simulink model "onboard_SSC_simscape"  (R2025b)
settings: Solver=ode23t  StartTime=0.0  StopTime=0.5  RelTol=1e-3
undefined symbols (not defined in the file): Second_OrderFilter_class, Vbat_ref
libraries: fl_lib x28, nesl_utility x14, ee_lib x8, mcbeeMathTransformLib x3, slpidlib x1, eeGeneralControl x1, batteryecm_lib x1, eeSinusoidalMeasurementV2 x1, simulink x1
(part 1 of 2)
settings Model: SimulationMode=accelerator  Creator=zxd3816  LastModifiedBy=agarcian
settings SolverCC: AlgebraicLoopSolver=TrustRegion
settings DataIOCC: SignalLogging=off  DSMLogging=off  ReturnWorkspaceOutputs=off
settings DebuggingCC: SaveWithParameterizedLinksMsg=none  UnconnectedInputMsg=warning  UnconnectedOutputMsg=warning  UnconnectedLineMsg=warning
settings ModelReferenceCC: EnableRefExpFcnMdlSchedulingChecks=on
settings RTWCC: GPUComputeCapability=3.5  DLArmComputeVersion=19.05

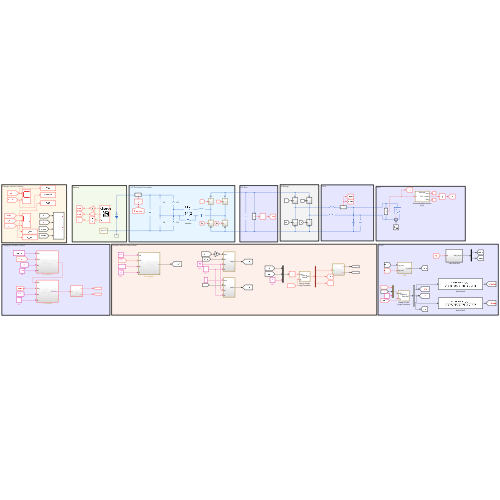
[thumbnail: Simulink's stored preview of the top-level diagram]
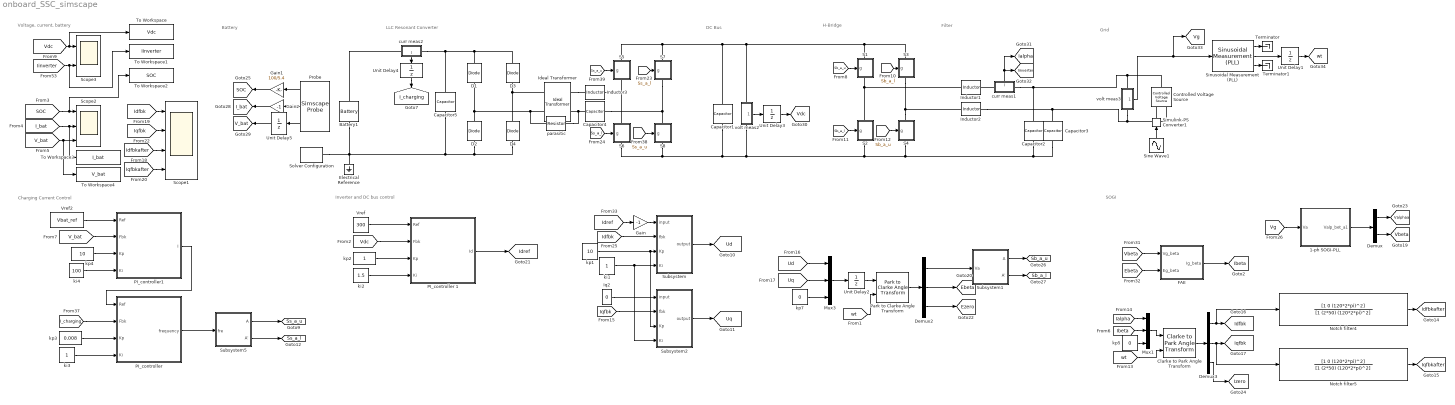
== system onboard_SSC_simscape ==
  note: Battery
  note: LLC Resonant Converter
  note: Charging Current Control
  note: SOGI
  note: Voltage, current, battery
  note: Inverter and DC bus control
  note: H-Bridge
  note: Filter
  note: DC Bus
  note: Grid
  1-ph SOGI-PLL : Subsystem
  Battery1 : batteryecm_lib/Battery  Vnom=100 V  prm_dir=simscape.enum.battery.prm_dir.disabled  R1_dis=2 Ohm  R1_ch=2 Ohm  R1=2 Ohm  prm_AH=simscape.enum.battery.prm_AH.finite  AH=5.4 A*hr  V1=95 V  AH1=0.54 A*hr  prm_R2=simscape.enum.battery.prm_R2.disabled  R2=2000 Ohm  Tmeas=298.15 K  charge_measurement_port=simscape.enum.battery.enable.no  prm_dyn=simscape.enum.battery.prm_dyn.off  Rp1=0.005 Ohm  tau1=30 s  Rp2=0.005 Ohm  tau2=30 s  Rp3=0.005 Ohm  tau3=30 s  Rp4=0.005 Ohm  tau4=30 s  Rp5=0.005 Ohm  tau5=30 s  prm_fade=simscape.enum.battery.prm_fade.disabled  N_fade=100  AH_fade=45 A*hr  R1_fade=2.02 Ohm  R1_ch_fade=2.02 Ohm  V1_fade=10.35 V  prm_age=simscape.enum.battery.prm_age.disabled  prm_age_OCV=simscape.enum.battery.prm_age_OCV.OCV  OCV_age=0.9  SOC_age=60  Tmeas_age=298.15 K  delta_time_age_vec=[0] d  temperature_age_vec=[273] K  OCV_scaling_age=2.2134e6  OCV_offset_age=1.632e6  temp_exp_age=0.515833569 V  t_exp_age=0.75  Vnom_T2=12 V  R1_T2=2.2 Ohm  R1_T2_dis=2.2 Ohm  R1_T2_ch=2.2 Ohm  V1_T2=11.4 V  R2_T2=2200 Ohm  Rp1_T2=0.005 Ohm  tau1_T2=30 s  Rp2_T2=0.005 Ohm  tau2_T2=30 s  Rp3_T2=0.005 Ohm  tau3_T2=30 s  Rp4_T2=0.005 Ohm  tau4_T2=30 s  Rp5_T2=0.005 Ohm  tau5_T2=30 s  Tmeas2=273.15 K  thermal_port=simscape.enum.thermaleffects.omit  thermal_mass=30000 J/K  i_specify=off  i_priority=None  i=0 A  i_nominal_specify=off  i_nominal_value=1  i_nominal_unit=A  v_specify=off  v_priority=None  v=0 V  v_nominal_specify=off  v_nominal_value=1  v_nominal_unit=V  charge_specify=on  charge_priority=High  charge=0.54 A*hr  charge_nominal_specify=off  charge_nominal_value=1  charge_nominal_unit=A*hr  num_cycles_specify=off  num_cycles_priority=High  num_cycles=0  num_cycles_nominal_specify=off  num_cycles_nominal_value=1  num_cycles_nominal_unit=1  temperature_specify=off  temperature_priority=High  temperature=298.15 K  temperature_nominal_specify=off  temperature_nominal_value=1  temperature_nominal_unit=K
  Capacitor1 : fl_lib/Electrical/Electrical Elements/Capacitor  c=500e-5 F  r=1e-9 Ohm  g=0 1/Ohm  i_specify=off  i_priority=None  i=0 A  i_nominal_specify=off  i_nominal_value=1  i_nominal_unit=A  v_specify=off  v_priority=None  v=0 V  v_nominal_specify=off  v_nominal_value=1  v_nominal_unit=V  vc_specify=off  vc_priority=High  vc=0 V  vc_nominal_specify=off  vc_nominal_value=1  vc_nominal_unit=V
  Capacitor2 : fl_lib/Electrical/Electrical Elements/Capacitor  c=60e-6 F  r=1e-9 Ohm  g=0 1/Ohm  i_specify=off  i_priority=None  i=0 A  i_nominal_specify=off  i_nominal_value=1  i_nominal_unit=A  v_specify=off  v_priority=None  v=0 V  v_nominal_specify=off  v_nominal_value=1  v_nominal_unit=V  vc_specify=off  vc_priority=High  vc=0 V  vc_nominal_specify=off  vc_nominal_value=1  vc_nominal_unit=V
  Capacitor3 : fl_lib/Electrical/Electrical Elements/Capacitor  c=60e-6 F  r=1e-9 Ohm  g=0 1/Ohm  i_specify=off  i_priority=None  i=0 A  i_nominal_specify=off  i_nominal_value=1  i_nominal_unit=A  v_specify=off  v_priority=None  v=0 V  v_nominal_specify=off  v_nominal_value=1  v_nominal_unit=V  vc_specify=off  vc_priority=High  vc=0 V  vc_nominal_specify=off  vc_nominal_value=1  vc_nominal_unit=V
  Capacitor4 : fl_lib/Electrical/Electrical Elements/Capacitor  c=110e-9 F  r=1e-6 Ohm  g=0 1/Ohm  i_specify=off  i_priority=None  i=0 A  i_nominal_specify=off  i_nominal_value=1  i_nominal_unit=A  v_specify=off  v_priority=None  v=0 V  v_nominal_specify=off  v_nominal_value=1  v_nominal_unit=V  vc_specify=off  vc_priority=High  vc=0 V  vc_nominal_specify=off  vc_nominal_value=1  vc_nominal_unit=V
  Capacitor5 : fl_lib/Electrical/Electrical Elements/Capacitor  c=500e-6 F  r=0 Ohm  g=0 1/Ohm  i_specify=off  i_priority=None  i=0 A  i_nominal_specify=off  i_nominal_value=1  i_nominal_unit=A  v_specify=off  v_priority=None  v=0 V  v_nominal_specify=off  v_nominal_value=1  v_nominal_unit=V  vc_specify=off  vc_priority=High  vc=0 V  vc_nominal_specify=off  vc_nominal_value=1  vc_nominal_unit=V
  Clarke to Park Angle Transform : mcbeeMathTransformLib/Clarke to Park Angle Transform  AxisAlignment=Q-axis  UseWithEmbedded=off  PhaseInput=Two inputs  ThetaInput=Sine and Cosine electrical position  AngleInput=Per-unit  N_points=1024
      settings: LibrarySourceBlock=|
      | ee_sl_lib/Mathematical
      | Transforms/Clarke to Park
      | Angle Transform
  Controlled Voltage Source : fl_lib/Electrical/Electrical Sources/Controlled Voltage Source
  D{1..4} (4 alike) : fl_lib/Electrical/Electrical Elements/Diode  Vf=0.8 V  Ron=0.001 Ohm  Goff=1/500 1/Ohm  i_specify=off  i_priority=None  i=0 A  i_nominal_specify=off  i_nominal_value=1  i_nominal_unit=A  v_specify=off  v_priority=None  v=0 V  v_nominal_specify=off  v_nominal_value=1  v_nominal_unit=V
  Demux : Demux  Outputs=2
  Demux2 : Demux  Outputs=3
  Demux3 : Demux  Outputs=3
  Electrical Reference : fl_lib/Electrical/Electrical Elements/Electrical Reference
  FAE : Subsystem
  Gain : Gain  Gain=-1
  Gain1 : Gain  Gain=100/5.4
  Gain2 : Gain  Gain=-1
  Ideal Transformer : fl_lib/Electrical/Electrical Elements/Ideal Transformer  n=1  i1_specify=off  i1_priority=None  i1=0 A  i1_nominal_specify=off  i1_nominal_value=1  i1_nominal_unit=A  v1_specify=off  v1_priority=None  v1=0 V  v1_nominal_specify=off  v1_nominal_value=1  v1_nominal_unit=V  i2_specify=off  i2_priority=None  i2=0 A  i2_nominal_specify=off  i2_nominal_value=1  i2_nominal_unit=A  v2_specify=off  v2_priority=None  v2=0 V  v2_nominal_specify=off  v2_nominal_value=1  v2_nominal_unit=V
  Inductor1 : fl_lib/Electrical/Electrical Elements/Inductor  l=3e-3 H  r=0.012 Ohm  g=0 1/Ohm  i_specify=off  i_priority=None  i=0 A  i_nominal_specify=off  i_nominal_value=1  i_nominal_unit=A  v_specify=off  v_priority=None  v=0 V  v_nominal_specify=off  v_nominal_value=1  v_nominal_unit=V  i_L_specify=off  i_L_priority=High  i_L=0 A  i_L_nominal_specify=off  i_L_nominal_value=1  i_L_nominal_unit=A
  Inductor2 : fl_lib/Electrical/Electrical Elements/Inductor  l=3e-3 H  r=0.012 Ohm  g=0 1/Ohm  i_specify=off  i_priority=None  i=0 A  i_nominal_specify=off  i_nominal_value=1  i_nominal_unit=A  v_specify=off  v_priority=None  v=0 V  v_nominal_specify=off  v_nominal_value=1  v_nominal_unit=V  i_L_specify=off  i_L_priority=High  i_L=0 A  i_L_nominal_specify=off  i_L_nominal_value=1  i_L_nominal_unit=A
  Inductor3 : fl_lib/Electrical/Electrical Elements/Inductor  l=21e-6 H  r=1e-6 Ohm  g=0 1/Ohm  i_specify=off  i_priority=None  i=0 A  i_nominal_specify=off  i_nominal_value=1  i_nominal_unit=A  v_specify=off  v_priority=None  v=0 V  v_nominal_specify=off  v_nominal_value=1  v_nominal_unit=V  i_L_specify=off  i_L_priority=High  i_L=0 A  i_L_nominal_specify=off  i_L_nominal_value=1  i_L_nominal_unit=A
  Iq2 : Constant  Value=0
  Mux1 : Mux  Inputs=3
  Mux3 : Mux  Inputs=3
  Notch filter4 : TransferFcn  Numerator=[1 0 (120*2*pi)^2]  Denominator=[1 (2*50) (120*2*pi)^2]
  Notch filter5 : TransferFcn  Numerator=[1 0 (120*2*pi)^2]  Denominator=[1 (2*50) (120*2*pi)^2]
  PI_controller : Subsystem
  PI_controller 1 : Subsystem
  PI_controller1 : Subsystem
  Park to Clarke Angle Transform : mcbeeMathTransformLib/Park to Clarke Angle Transform  AxisAlignment=Q-axis  UseWithEmbedded=off  PhaseInput=Two inputs  ThetaInput=Sine and Cosine electrical position  AngleInput=Per-unit  N_points=1024
      settings: LibrarySourceBlock=|
      | ee_sl_lib/Mathematical
      | Transforms/Park to Clarke
      | Angle Transform
  Probe : SimscapeProbe  BoundBlock=1503  Variables="{\"charge\":{\"Probing\":\"ON\"},\"i\":{\"Probing\":\"ON\"},\"v\":{\"Probing\":\"ON\"}}"
  S1 : Subsystem
      settings: PortSchema="{\"entries\":[{\"content\":{\"sides\":[{\"content\":{\"connectorIds\":[\"In1\"]},\"type\":\"ConnectorPlacement.EquallySpacedRectSide\",\"uuid\":\"60fc8352-b056-4a1d-84e9-807da1ce3c88\"},{\"content\":{\"side\":\"RIGHT\"},\"type\":\"ConnectorPlacement.EquallySpacedRectSide\",\"uuid\":\"4f85bb6a-64c7-4bda-b651-7e84ba390faf\"},{\"content\":{\"connectorIds\":[\"LConn1\"],\"side\":\"TOP\"},\"type\":\"ConnectorPlacement.EquallySpacedRectSide\",\"uuid\":\"49a2dfe1-7dda-4371-a15a-7ad00d7eb6fd\"},{\"content\":{\"connectorIds\":[\"RConn1\"],\"side\":\"BOTTOM\"},\"type\":\"ConnectorPlacement.EquallySpacedRectSide\",\"uuid\":\"2b076144-f23a-4c54-b109-69957c2c042c\"}]},\"type\":\"ConnectorPlacement.EquallySpacedConnector\",\"uuid\":\"c494b7b1-a248-4760-aec7-aedba1239c75\"}],\"packageUris\":[\"http://schema.mathworks.com/mf0/Connector/R2020b\"],\"version\":\"1.0\"}"
  S2 : Subsystem
      settings: PortSchema="{\"entries\":[{\"content\":{\"sides\":[{\"content\":{\"connectorIds\":[\"In1\"]},\"type\":\"ConnectorPlacement.EquallySpacedRectSide\",\"uuid\":\"60fc8352-b056-4a1d-84e9-807da1ce3c88\"},{\"content\":{\"side\":\"RIGHT\"},\"type\":\"ConnectorPlacement.EquallySpacedRectSide\",\"uuid\":\"4f85bb6a-64c7-4bda-b651-7e84ba390faf\"},{\"content\":{\"connectorIds\":[\"LConn1\"],\"side\":\"TOP\"},\"type\":\"ConnectorPlacement.EquallySpacedRectSide\",\"uuid\":\"49a2dfe1-7dda-4371-a15a-7ad00d7eb6fd\"},{\"content\":{\"connectorIds\":[\"RConn1\"],\"side\":\"BOTTOM\"},\"type\":\"ConnectorPlacement.EquallySpacedRectSide\",\"uuid\":\"2b076144-f23a-4c54-b109-69957c2c042c\"}]},\"type\":\"ConnectorPlacement.EquallySpacedConnector\",\"uuid\":\"c494b7b1-a248-4760-aec7-aedba1239c75\"}],\"packageUris\":[\"http://schema.mathworks.com/mf0/Connector/R2020b\"],\"version\":\"1.0\"}"
  S3 : Subsystem
      settings: PortSchema="{\"entries\":[{\"content\":{\"sides\":[{\"content\":{\"connectorIds\":[\"In1\"]},\"type\":\"ConnectorPlacement.EquallySpacedRectSide\",\"uuid\":\"60fc8352-b056-4a1d-84e9-807da1ce3c88\"},{\"content\":{\"side\":\"RIGHT\"},\"type\":\"ConnectorPlacement.EquallySpacedRectSide\",\"uuid\":\"4f85bb6a-64c7-4bda-b651-7e84ba390faf\"},{\"content\":{\"connectorIds\":[\"LConn1\"],\"side\":\"TOP\"},\"type\":\"ConnectorPlacement.EquallySpacedRectSide\",\"uuid\":\"49a2dfe1-7dda-4371-a15a-7ad00d7eb6fd\"},{\"content\":{\"connectorIds\":[\"RConn1\"],\"side\":\"BOTTOM\"},\"type\":\"ConnectorPlacement.EquallySpacedRectSide\",\"uuid\":\"2b076144-f23a-4c54-b109-69957c2c042c\"}]},\"type\":\"ConnectorPlacement.EquallySpacedConnector\",\"uuid\":\"c494b7b1-a248-4760-aec7-aedba1239c75\"}],\"packageUris\":[\"http://schema.mathworks.com/mf0/Connector/R2020b\"],\"version\":\"1.0\"}"
  S4 : Subsystem
      settings: PortSchema="{\"entries\":[{\"content\":{\"sides\":[{\"content\":{\"connectorIds\":[\"In1\"]},\"type\":\"ConnectorPlacement.EquallySpacedRectSide\",\"uuid\":\"60fc8352-b056-4a1d-84e9-807da1ce3c88\"},{\"content\":{\"side\":\"RIGHT\"},\"type\":\"ConnectorPlacement.EquallySpacedRectSide\",\"uuid\":\"4f85bb6a-64c7-4bda-b651-7e84ba390faf\"},{\"content\":{\"connectorIds\":[\"LConn1\"],\"side\":\"TOP\"},\"type\":\"ConnectorPlacement.EquallySpacedRectSide\",\"uuid\":\"49a2dfe1-7dda-4371-a15a-7ad00d7eb6fd\"},{\"content\":{\"connectorIds\":[\"RConn1\"],\"side\":\"BOTTOM\"},\"type\":\"ConnectorPlacement.EquallySpacedRectSide\",\"uuid\":\"2b076144-f23a-4c54-b109-69957c2c042c\"}]},\"type\":\"ConnectorPlacement.EquallySpacedConnector\",\"uuid\":\"c494b7b1-a248-4760-aec7-aedba1239c75\"}],\"packageUris\":[\"http://schema.mathworks.com/mf0/Connector/R2020b\"],\"version\":\"1.0\"}"
  S5 : Subsystem
      settings: PortSchema="{\"entries\":[{\"content\":{\"sides\":[{\"content\":{\"connectorIds\":[\"In1\"]},\"type\":\"ConnectorPlacement.EquallySpacedRectSide\",\"uuid\":\"60fc8352-b056-4a1d-84e9-807da1ce3c88\"},{\"content\":{\"side\":\"RIGHT\"},\"type\":\"ConnectorPlacement.EquallySpacedRectSide\",\"uuid\":\"4f85bb6a-64c7-4bda-b651-7e84ba390faf\"},{\"content\":{\"connectorIds\":[\"LConn1\"],\"side\":\"TOP\"},\"type\":\"ConnectorPlacement.EquallySpacedRectSide\",\"uuid\":\"49a2dfe1-7dda-4371-a15a-7ad00d7eb6fd\"},{\"content\":{\"connectorIds\":[\"RConn1\"],\"side\":\"BOTTOM\"},\"type\":\"ConnectorPlacement.EquallySpacedRectSide\",\"uuid\":\"2b076144-f23a-4c54-b109-69957c2c042c\"}]},\"type\":\"ConnectorPlacement.EquallySpacedConnector\",\"uuid\":\"c494b7b1-a248-4760-aec7-aedba1239c75\"}],\"packageUris\":[\"http://schema.mathworks.com/mf0/Connector/R2020b\"],\"version\":\"1.0\"}"
  S6 : Subsystem
      settings: PortSchema="{\"entries\":[{\"content\":{\"sides\":[{\"content\":{\"connectorIds\":[\"In1\"]},\"type\":\"ConnectorPlacement.EquallySpacedRectSide\",\"uuid\":\"60fc8352-b056-4a1d-84e9-807da1ce3c88\"},{\"content\":{\"side\":\"RIGHT\"},\"type\":\"ConnectorPlacement.EquallySpacedRectSide\",\"uuid\":\"4f85bb6a-64c7-4bda-b651-7e84ba390faf\"},{\"content\":{\"connectorIds\":[\"LConn1\"],\"side\":\"TOP\"},\"type\":\"ConnectorPlacement.EquallySpacedRectSide\",\"uuid\":\"49a2dfe1-7dda-4371-a15a-7ad00d7eb6fd\"},{\"content\":{\"connectorIds\":[\"RConn1\"],\"side\":\"BOTTOM\"},\"type\":\"ConnectorPlacement.EquallySpacedRectSide\",\"uuid\":\"2b076144-f23a-4c54-b109-69957c2c042c\"}]},\"type\":\"ConnectorPlacement.EquallySpacedConnector\",\"uuid\":\"c494b7b1-a248-4760-aec7-aedba1239c75\"}],\"packageUris\":[\"http://schema.mathworks.com/mf0/Connector/R2020b\"],\"version\":\"1.0\"}"
  S7 : Subsystem
      settings: PortSchema="{\"entries\":[{\"content\":{\"sides\":[{\"content\":{\"connectorIds\":[\"In1\"]},\"type\":\"ConnectorPlacement.EquallySpacedRectSide\",\"uuid\":\"60fc8352-b056-4a1d-84e9-807da1ce3c88\"},{\"content\":{\"side\":\"RIGHT\"},\"type\":\"ConnectorPlacement.EquallySpacedRectSide\",\"uuid\":\"4f85bb6a-64c7-4bda-b651-7e84ba390faf\"},{\"content\":{\"connectorIds\":[\"LConn1\"],\"side\":\"TOP\"},\"type\":\"ConnectorPlacement.EquallySpacedRectSide\",\"uuid\":\"49a2dfe1-7dda-4371-a15a-7ad00d7eb6fd\"},{\"content\":{\"connectorIds\":[\"RConn1\"],\"side\":\"BOTTOM\"},\"type\":\"ConnectorPlacement.EquallySpacedRectSide\",\"uuid\":\"2b076144-f23a-4c54-b109-69957c2c042c\"}]},\"type\":\"ConnectorPlacement.EquallySpacedConnector\",\"uuid\":\"c494b7b1-a248-4760-aec7-aedba1239c75\"}],\"packageUris\":[\"http://schema.mathworks.com/mf0/Connector/R2020b\"],\"version\":\"1.0\"}"
  S8 : Subsystem
      settings: PortSchema="{\"entries\":[{\"content\":{\"sides\":[{\"content\":{\"connectorIds\":[\"In1\"]},\"type\":\"ConnectorPlacement.EquallySpacedRectSide\",\"uuid\":\"60fc8352-b056-4a1d-84e9-807da1ce3c88\"},{\"content\":{\"side\":\"RIGHT\"},\"type\":\"ConnectorPlacement.EquallySpacedRectSide\",\"uuid\":\"4f85bb6a-64c7-4bda-b651-7e84ba390faf\"},{\"content\":{\"connectorIds\":[\"LConn1\"],\"side\":\"TOP\"},\"type\":\"ConnectorPlacement.EquallySpacedRectSide\",\"uuid\":\"49a2dfe1-7dda-4371-a15a-7ad00d7eb6fd\"},{\"content\":{\"connectorIds\":[\"RConn1\"],\"side\":\"BOTTOM\"},\"type\":\"ConnectorPlacement.EquallySpacedRectSide\",\"uuid\":\"2b076144-f23a-4c54-b109-69957c2c042c\"}]},\"type\":\"ConnectorPlacement.EquallySpacedConnector\",\"uuid\":\"c494b7b1-a248-4760-aec7-aedba1239c75\"}],\"packageUris\":[\"http://schema.mathworks.com/mf0/Connector/R2020b\"],\"version\":\"1.0\"}"
  Scope1 : Scope  NumInputPorts=4
      settings: ActiveDisplayYMinimum=-174.13299  ActiveDisplayYMaximum=150.39718
  Scope2 : Scope  NumInputPorts=3
      settings: ActiveDisplayYMinimum=9.9934066794791612  ActiveDisplayYMaximum=10.056826198144963
  Scope3 : Scope  NumInputPorts=2
      settings: ActiveDisplayYMinimum=-38.68725  ActiveDisplayYMaximum=348.18522  DataLoggingVariableName=ScopeData3
  Simulink-PS Converter1 : nesl_utility/Simulink-PS Converter  PhysicalDomain=network_engine_domain  SubClassName=ps_input  LeftPortType=input  RightPortType=output  PseudoPeriodic=off  Frequencies=[]  NoiseDistribution=none  NoiseParameters=[]  Unit=1  AffineConversion=off  FilteringAndDerivatives=provide  SimscapeFilterOrder=1  InputFilterTimeConstant=0.001  UdotUserProvided=0
  Sine Wave1 : Sin  Amplitude=169.7  Frequency=60*2*pi  SampleTime=0
  Sinusoidal Measurement (PLL) : eeSinusoidalMeasurementV2/Sinusoidal Measurement (PLL)  Ki_PD=3200  Kp_LF=180  Ki_LF=3200  F0=60  Theta0=0  Mag0=1  Ts=-1
      settings: LibrarySourceBlock=|
      | ee_sl_lib/Measurements/Sinusoidal Measurement
      | (PLL)
  Solver Configuration : nesl_utility/Solver Configuration  PhysicalDomain=network_engine_domain  SubClassName=solver  LeftPortType=input  RightPortType=generic  Tones=[]  Harmonics=[]  SimulateNoise=off  Profile=off  UseLocalSampling=off  EnableSwitchedLinearOptims=on  FrequencyDomain=off  UseCCode=off  RelTol=0.001  AbsTol=0.001  MinStep=1e-09  ToWorkspace=off  RevertToSquareIcSolve=off  NumHomotopyIterations=100  PhasorMode=off  PhasorModeNumHarmonics=1  ConsistencySolver=NEWTON_XTOL_AFTER_FTOL  IndexReductionMethod=DerivativeReplacement  DoDC=off  ResidualTolerance=1e-09  ConsistencyTolSource=GLOBAL  ConsistencyAbsTol=0.001  ConsistencyRelTol=0.001  ConsistencyTolFactor=0.001  UseLocalSolver=on  LocalSolverChoice=NE_PARTITIONING_ADVANCER  ResolveIndetEquations=off  FunctionEvalNumThread=1  LocalSolverSampleTime=1e-7  DoFixedCost=off  MaxNonlinIter=2  MaxModeIter=2  ComputeImpulses=off  ImpulseIterations=2  LinearAlgebra=auto  LinearAlgebraNumThread=0  EquationFormulation=NE_TIME_EF  DelaysMemoryBudget=1024  AutomaticFiltering=off  FilteringTimeConstant=0.001  PartitionStorageMethod=AS_NEEDED  PartitionMemoryBudget=1024  PartitionMethod=ROBUST  MultibodyUseLocalSolver=off  MultibodyLocalSolverChoice=ODE1  MultibodyLocalSolverSampleTime=0.001
  Subsystem : Subsystem
  Subsystem1 : Subsystem
  Subsystem2 : Subsystem
  Subsystem5 : Subsystem
  Terminator : Terminator
  Terminator1 : Terminator
  To Workspace : ToWorkspace  VariableName=Vdc  SampleTime=-1
  To Workspace1 : ToWorkspace  VariableName=Iinverter  SampleTime=-1
  To Workspace2 : ToWorkspace  VariableName=SOC  SampleTime=-1
  To Workspace3 : ToWorkspace  VariableName=I_bat  SampleTime=-1
  To Workspace4 : ToWorkspace  VariableName=V_bat  SampleTime=-1
  Unit Delay{1..5} (5 alike) : UnitDelay  SampleTime=-1  HasFrameUpgradeWarning=on
  Vref : Constant  Value=300
  Vref2 : Constant  Value=Vbat_ref
  curr meas1 : Subsystem
      settings: PortSchema="{\"entries\":[{\"content\":{\"sides\":[{\"content\":{\"connectorIds\":[\"LConn1\"]},\"type\":\"ConnectorPlacement.EquallySpacedRectSide\",\"uuid\":\"624dd8c9-1efa-425a-b23f-9e7d392e4567\"},{\"content\":{\"connectorIds\":[\"RConn1\"],\"side\":\"RIGHT\"},\"type\":\"ConnectorPlacement.EquallySpacedRectSide\",\"uuid\":\"c564bb74-22a6-4c48-884d-57ae53c7e586\"},{\"content\":{\"connectorIds\":[\"Out1\"],\"side\":\"TOP\"},\"type\":\"ConnectorPlacement.EquallySpacedRectSide\",\"uuid\":\"df3a0756-8bf4-4498-aa4e-0bb1b4f3eded\"}]},\"type\":\"ConnectorPlacement.EquallySpacedConnector\",\"uuid\":\"9eff73ec-b3ab-492c-96fa-8ca694a66385\"}],\"packageUris\":[\"http://schema.mathworks.com/mf0/Connector/R2020b\"],\"version\":\"1.0\"}"
  curr meas2 : Subsystem
      settings: PortSchema="{\"entries\":[{\"content\":{\"sides\":[{\"content\":{\"connectorIds\":[\"LConn1\"]},\"type\":\"ConnectorPlacement.EquallySpacedRectSide\",\"uuid\":\"624dd8c9-1efa-425a-b23f-9e7d392e4567\"},{\"content\":{\"connectorIds\":[\"RConn1\"],\"side\":\"RIGHT\"},\"type\":\"ConnectorPlacement.EquallySpacedRectSide\",\"uuid\":\"c564bb74-22a6-4c48-884d-57ae53c7e586\"},{\"content\":{\"connectorIds\":[\"Out1\"],\"side\":\"TOP\"},\"type\":\"ConnectorPlacement.EquallySpacedRectSide\",\"uuid\":\"df3a0756-8bf4-4498-aa4e-0bb1b4f3eded\"}]},\"type\":\"ConnectorPlacement.EquallySpacedConnector\",\"uuid\":\"9eff73ec-b3ab-492c-96fa-8ca694a66385\"}],\"packageUris\":[\"http://schema.mathworks.com/mf0/Connector/R2020b\"],\"version\":\"1.0\"}"
  ki1 : Constant
  ki2 : Constant  Value=1.5
  ki3 : Constant
  ki4 : Constant  Value=100
  kp1 : Constant  Value=10
  kp2 : Constant
  kp3 : Constant  Value=0.008
  kp4 : Constant  Value=10
  kp5 : Constant  Value=0
  kp7 : Constant  Value=0
  parasitic : fl_lib/Electrical/Electrical Elements/Resistor  R=1e8 Ohm  i_specify=off  i_priority=None  i=0 A  i_nominal_specify=off  i_nominal_value=1  i_nominal_unit=A  v_specify=off  v_priority=None  v=0 V  v_nominal_specify=off  v_nominal_value=1  v_nominal_unit=V
  volt meas2 : Subsystem
      settings: PortSchema="{\"entries\":[{\"content\":{\"sides\":[{\"content\":{},\"type\":\"ConnectorPlacement.EquallySpacedRectSide\",\"uuid\":\"624dd8c9-1efa-425a-b23f-9e7d392e4567\"},{\"content\":{\"connectorIds\":[\"Out1\"],\"side\":\"RIGHT\"},\"type\":\"ConnectorPlacement.EquallySpacedRectSide\",\"uuid\":\"c564bb74-22a6-4c48-884d-57ae53c7e586\"},{\"content\":{\"connectorIds\":[\"LConn1\"],\"side\":\"TOP\"},\"type\":\"ConnectorPlacement.EquallySpacedRectSide\",\"uuid\":\"df3a0756-8bf4-4498-aa4e-0bb1b4f3eded\"},{\"content\":{\"connectorIds\":[\"RConn1\"],\"side\":\"BOTTOM\"},\"type\":\"ConnectorPlacement.EquallySpacedRectSide\",\"uuid\":\"6b8e9540-8d6f-4bd3-bf1f-20eb25478a8e\"}]},\"type\":\"ConnectorPlacement.EquallySpacedConnector\",\"uuid\":\"9eff73ec-b3ab-492c-96fa-8ca694a66385\"}],\"packageUris\":[\"http://schema.mathworks.com/mf0/Connector/R2020b\"],\"version\":\"1.0\"}"
  volt meas3 : Subsystem
      settings: PortSchema="{\"entries\":[{\"content\":{\"sides\":[{\"content\":{},\"type\":\"ConnectorPlacement.EquallySpacedRectSide\",\"uuid\":\"624dd8c9-1efa-425a-b23f-9e7d392e4567\"},{\"content\":{\"connectorIds\":[\"Out1\"],\"side\":\"RIGHT\"},\"type\":\"ConnectorPlacement.EquallySpacedRectSide\",\"uuid\":\"c564bb74-22a6-4c48-884d-57ae53c7e586\"},{\"content\":{\"connectorIds\":[\"LConn1\"],\"side\":\"TOP\"},\"type\":\"ConnectorPlacement.EquallySpacedRectSide\",\"uuid\":\"df3a0756-8bf4-4498-aa4e-0bb1b4f3eded\"},{\"content\":{\"connectorIds\":[\"RConn1\"],\"side\":\"BOTTOM\"},\"type\":\"ConnectorPlacement.EquallySpacedRectSide\",\"uuid\":\"6b8e9540-8d6f-4bd3-bf1f-20eb25478a8e\"}]},\"type\":\"ConnectorPlacement.EquallySpacedConnector\",\"uuid\":\"9eff73ec-b3ab-492c-96fa-8ca694a66385\"}],\"packageUris\":[\"http://schema.mathworks.com/mf0/Connector/R2020b\"],\"version\":\"1.0\"}"
  tag scope: Ebeta=global, Ezero=global, I_bat=global, I_charging=global, Ialpha=global, Ibeta=global, Idfbk=global, Idfbkafter=global, Idref=global, Iinverter=global, Iqfbk=global, Iqfbkafter=global, Izero=global, SOC=global, Sb_a_l=global, Sb_a_u=global, Ss_a_l=global, Ss_a_u=global, Ud=global, Uq=global, V_bat=global, Valphaa=global, Vbeta=global, Vdc=global, Vg=global, wt=global
  wires:
  [Iqfbk] -> Scope1/2
  [Idfbk] -> Scope1/1
  [Vdc] -> To Workspace/1, Scope3/1
  [Iinverter] -> To Workspace1/1, Scope3/2
  Demux2/3 -> [Ezero]
  Subsystem/1(output) -> [Ud]
  kp1/1 -> Subsystem2/3(Kp), Subsystem/3(Kp)
  Subsystem2/1(output) -> [Uq]
  ki1/1 -> Subsystem2/4(Ki), Subsystem/4(Ki)
  kp2/1 -> PI_controller 1/3(Kp)
  ki2/1 -> PI_controller 1/4(Ki)
  Vref/1 -> PI_controller 1/1(Ref)
  [Vdc] -> PI_controller 1/2(Fbk)
  Iq2/1 -> Subsystem2/1(input)
  [Iqfbk] -> Subsystem2/2(fbk)
  Demux2/1 -> Subsystem1/1(Va)
  [Idfbk] -> Subsystem/2(fbk)
  Mux3/1 -> Unit Delay2/1
  [Ud] -> Mux3/1
  [Uq] -> Mux3/2
  kp7/1 -> Mux3/3
  [wt] -> Park to Clarke Angle Transform/2
  Park to Clarke Angle Transform/1 -> Demux2/1
  Demux3/1 -> Notch filter4/1, [Idfbk]
  Notch filter4/1 -> [Idfbkafter]
  Clarke to Park Angle Transform/1 -> Demux3/1
  Notch filter5/1 -> [Iqfbkafter]
  [wt] -> Clarke to Park Angle Transform/2
  Demux3/2 -> Notch filter5/1, [Iqfbk]
  Mux1/1 -> Clarke to Park Angle Transform/1
  [Ialpha] -> Mux1/1
  1-ph SOGI-PLL/1(Valp_bet_a1) -> Demux/1
  FAE/1(Ig_beta) -> [Ibeta]
  [Ibeta] -> Mux1/2
  [Idfbkafter] -> Scope1/3
  [Iqfbkafter] -> Scope1/4
  [Vg] -> 1-ph SOGI-PLL/1(Va)
  Demux/2 -> [Vbeta]
  [Vbeta] -> FAE/1(Vg_beta)
  Demux2/2 -> [Ebeta]
  [Ebeta] -> FAE/2(Eg_beta)
  PI_controller 1/1(Id) -> [Idref]
  Demux/1 -> [Valphaa]
  Demux3/3 -> [Izero]
  Gain/1 -> Subsystem/1(input)
  Subsystem1/1(A) -> [Sb_a_u]
  Subsystem1/2(A') -> [Sb_a_l]
  [Idref] -> Gain/1
  Subsystem5/1(A) -> [Ss_a_u]
  Subsystem5/2(A') -> [Ss_a_l]
  PI_controller/1(frequency) -> Subsystem5/1(fre)
  kp3/1 -> PI_controller/3(Kp)
  ki3/1 -> PI_controller/4(Ki)
  [I_charging] -> PI_controller/2(Fbk)
  [SOC] -> To Workspace2/1, Scope2/1
  [I_bat] -> To Workspace3/1, Scope2/2
  [V_bat] -> To Workspace4/1, Scope2/3
  Vref2/1 -> PI_controller1/1(Ref)
  [V_bat] -> PI_controller1/2(Fbk)
  kp4/1 -> PI_controller1/3(Kp)
  ki4/1 -> PI_controller1/4(Ki)
  PI_controller1/1(I) -> PI_controller/1(Ref)
  volt meas2/1(V) -> Unit Delay3/1
  Sinusoidal Measurement (PLL)/2 -> Unit Delay1/1
  Sinusoidal Measurement (PLL)/1 -> Terminator/1
  Unit Delay3/1 -> [Vdc]
  [Sb_a_u] -> S4/1(g)
  curr meas1/1(I) -> [Iinverter], [Ialpha]
  Sinusoidal Measurement (PLL)/3 -> Terminator1/1
  [Sb_a_u] -> S1/1(g)
  [Sb_a_l] -> S3/1(g)
  Unit Delay1/1 -> [wt]
  Sine Wave1/1 -> Simulink-PS Converter1/1
  volt meas3/1(V) -> Sinusoidal Measurement (PLL)/1, [Vg]
  [Sb_a_l] -> S2/1(g)
  [Ss_a_l] -> S6/1(g)
  [Ss_a_l] -> S7/1(g)
  [Ss_a_u] -> S5/1(g)
  [Ss_a_u] -> S8/1(g)
  curr meas2/1(I) -> Unit Delay4/1
  Probe/1 -> Gain1/1
  Probe/3 -> Unit Delay5/1
  Gain1/1 -> [SOC]
  kp5/1 -> Mux1/3
  Unit Delay2/1 -> Park to Clarke Angle Transform/1
  Unit Delay4/1 -> [I_charging]
  Unit Delay5/1 -> [V_bat]
  Probe/2 -> Gain2/1
  Gain2/1 -> [I_bat]
  connections:
  S7/LConn1 -- volt meas2/LConn1 -- S3/LConn1 -- S1/LConn1 -- Capacitor1/LConn1 -- S5/LConn1
  Capacitor2/RConn1 -- volt meas2/RConn1 -- Capacitor1/RConn1 -- S8/RConn1 -- S6/RConn1 -- S2/RConn1 -- S4/RConn1 -- Capacitor3/RConn1
  Capacitor2/LConn1 -- curr meas1/RConn1 -- Controlled Voltage Source/LConn1 -- volt meas3/LConn1
  Controlled Voltage Source/RConn2 -- volt meas3/RConn1 -- Inductor2/RConn1 -- Capacitor3/LConn1
  Inductor1/LConn1 -- S2/LConn1 -- S1/RConn1
  S4/LConn1 -- S3/RConn1 -- Inductor2/LConn1
  Simulink-PS Converter1/RConn1 -- Controlled Voltage Source/RConn1
  curr meas1/LConn1 -- Inductor1/RConn1
  Ideal Transformer/RConn1 -- Inductor3/LConn1
  Ideal Transformer/RConn2 -- parasitic/RConn1 -- Capacitor4/LConn1
  S6/LConn1 -- Inductor3/RConn1 -- S5/RConn1
  S7/RConn1 -- S8/LConn1 -- Capacitor4/RConn1
  D2/RConn1 -- parasitic/LConn1 -- Ideal Transformer/LConn2 -- D1/LConn1
  D4/RConn1 -- Ideal Transformer/LConn1 -- D3/LConn1
  D3/RConn1 -- Capacitor5/LConn1 -- curr meas2/LConn1 -- D1/RConn1
  D4/LConn1 -- D2/LConn1 -- Electrical Reference/LConn1 -- Battery1/RConn1 -- Solver Configuration/RConn1 -- Capacitor5/RConn1
  Battery1/LConn1 -- curr meas2/RConn1

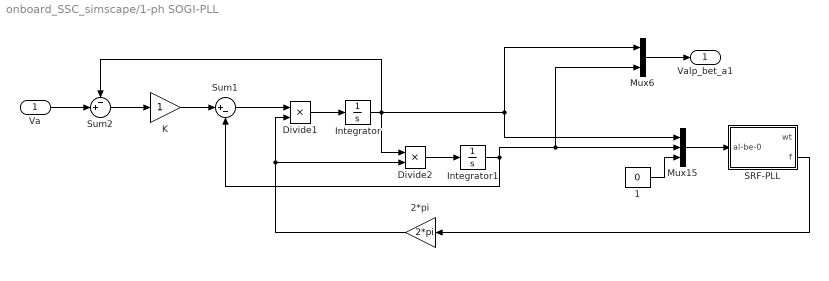
== system onboard_SSC_simscape/1-ph SOGI-PLL ==
  Va : Inport
  1 : Constant  Value=0
  2*pi : Gain  Gain=2*pi
  Divide1 : Product  Inputs=**
  Divide2 : Product  Inputs=**
  Integrator : Integrator
  Integrator1 : Integrator
  K : Gain
  Mux15 : Mux  Inputs=3
  Mux6 : Mux  Inputs=2
  SRF-PLL : Subsystem
  Sum1 : Sum  Inputs=|+-
  Sum2 : Sum  Inputs=-+|
  Valp_bet_a1 : Outport
  wires:
  Divide1/1 -> Integrator/1
  Sum1/1 -> Divide1/1
  K/1 -> Sum1/1
  Sum2/1 -> K/1
  Integrator/1 -> Sum2/1, Divide2/1, Mux15/1, Mux6/1
  Divide2/1 -> Integrator1/1
  Integrator1/1 -> Sum1/2, Mux6/2, Mux15/2
  Va/1 -> Sum2/2
  1/1 -> Mux15/3
  Mux15/1 -> SRF-PLL/1(al-be-0)
  2*pi/1 -> Divide2/2, Divide1/2
  SRF-PLL/2(f) -> 2*pi/1
  Mux6/1 -> Valp_bet_a1/1

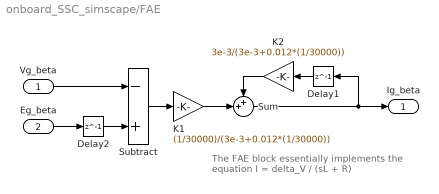
== system onboard_SSC_simscape/FAE ==
  note: The FAE block essentially implements the equation I = delta_V / (sL + R)
  Vg_beta : Inport
  Eg_beta : Inport  Port=2
  Delay1 : Delay  DelayLength=1
  Delay2 : Delay  DelayLength=1
  K1 : Gain  Gain=(1/30000)/(3e-3+0.012*(1/30000))
  K2 : Gain  Gain=3e-3/(3e-3+0.012*(1/30000))
  Subtract : Sum  Inputs=-+
  Sum : Sum  Inputs=++|
  Ig_beta : Outport
  wires:
  Eg_beta/1 -> Delay2/1
  Delay2/1 -> Subtract/2
  Sum/1 -> Ig_beta/1, Delay1/1
  K2/1 -> Sum/1
  Delay1/1 -> K2/1
  K1/1 -> Sum/2
  Subtract/1 -> K1/1
  Vg_beta/1 -> Subtract/1

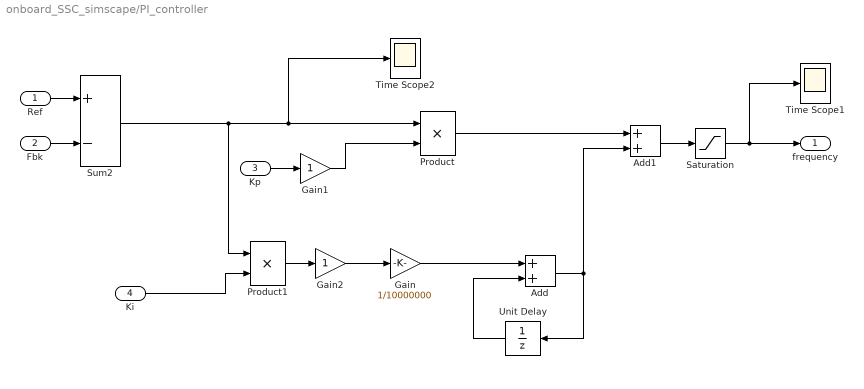
== system onboard_SSC_simscape/PI_controller ==
  Ref : Inport
  Fbk : Inport  Port=2
  Kp : Inport  Port=3
  Ki : Inport  Port=4
  Add : Sum
  Add1 : Sum
  Gain : Gain  Gain=1/10000000
  Gain1 : Gain
  Gain2 : Gain
  Product : Product  OutDataTypeStr=Inherit: Same as first input
  Product1 : Product  OutDataTypeStr=Inherit: Same as first input
  Saturation : Saturate  UpperLimit=1  LowerLimit=0.5  LinearizeAsGain=off  ZeroCross=off
  Sum2 : Sum  Inputs=+-
  Time Scope1 : Scope
      settings: TimeUnits=Metric (based on Time Span)  ActiveDisplayYMinimum=0.5433  ActiveDisplayYMaximum=1.0015  YLabel=Amplitude  DataLoggingVariableName=ScopeData5
  Time Scope2 : Scope
      settings: TimeUnits=Metric (based on Time Span)  ActiveDisplayYMinimum=-48.22028  ActiveDisplayYMaximum=227.58003  YLabel=Amplitude  DataLoggingVariableName=ScopeData6
  Unit Delay : UnitDelay  InitialCondition=0.9  SampleTime=-1  HasFrameUpgradeWarning=on
  frequency : Outport
  wires:
  Fbk/1 -> Sum2/2
  Ref/1 -> Sum2/1
  Product1/1 -> Gain2/1
  Add/1 -> Unit Delay/1, Add1/2
  Product/1 -> Add1/1
  Gain/1 -> Add/1
  Unit Delay/1 -> Add/2
  Ki/1 -> Product1/2
  Gain2/1 -> Gain/1
  Add1/1 -> Saturation/1
  Saturation/1 -> Time Scope1/1, frequency/1
  Kp/1 -> Gain1/1
  Gain1/1 -> Product/2
  Sum2/1 -> Product1/1, Time Scope2/1, Product/1

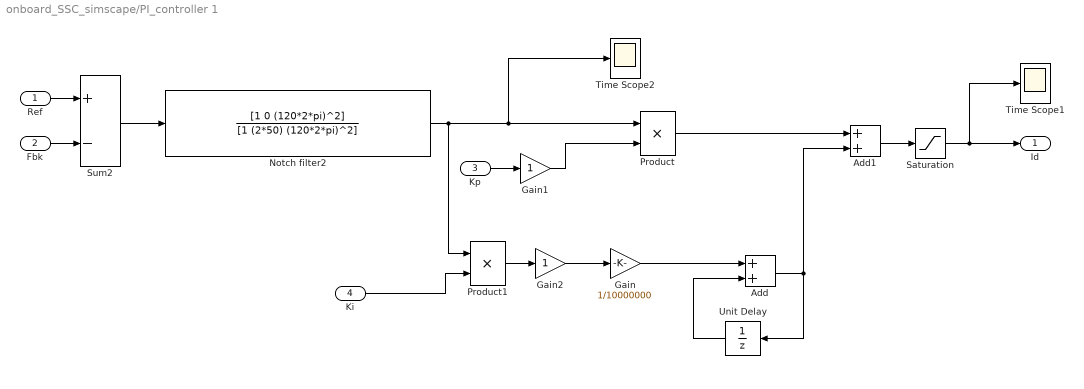
== system onboard_SSC_simscape/PI_controller 1 ==
  Ref : Inport
  Fbk : Inport  Port=2
  Kp : Inport  Port=3
  Ki : Inport  Port=4
  Add : Sum
  Add1 : Sum
  Gain : Gain  Gain=1/10000000
  Gain1 : Gain
  Gain2 : Gain
  Notch filter2 : TransferFcn  Numerator=[1 0 (120*2*pi)^2]  Denominator=[1 (2*50) (120*2*pi)^2]
  Product : Product  OutDataTypeStr=Inherit: Same as first input
  Product1 : Product  OutDataTypeStr=Inherit: Same as first input
  Saturation : Saturate  UpperLimit=100  LowerLimit=-100  LinearizeAsGain=off  ZeroCross=off
  Sum2 : Sum  Inputs=+-
  Time Scope1 : Scope
      settings: TimeUnits=Metric (based on Time Span)  ActiveDisplayYMinimum=-62.5  ActiveDisplayYMaximum=62.5  YLabel=Amplitude  DataLoggingVariableName=ScopeData5
  Time Scope2 : Scope
      settings: TimeUnits=Metric (based on Time Span)  ActiveDisplayYMinimum=-48.22028  ActiveDisplayYMaximum=227.58003  YLabel=Amplitude  DataLoggingVariableName=ScopeData6
  Unit Delay : UnitDelay  SampleTime=-1  HasFrameUpgradeWarning=on
  Id : Outport
  wires:
  Fbk/1 -> Sum2/2
  Ref/1 -> Sum2/1
  Product1/1 -> Gain2/1
  Add/1 -> Unit Delay/1, Add1/2
  Product/1 -> Add1/1
  Gain/1 -> Add/1
  Unit Delay/1 -> Add/2
  Ki/1 -> Product1/2
  Gain2/1 -> Gain/1
  Add1/1 -> Saturation/1
  Saturation/1 -> Time Scope1/1, Id/1
  Kp/1 -> Gain1/1
  Gain1/1 -> Product/2
  Sum2/1 -> Notch filter2/1
  Notch filter2/1 -> Product1/1, Time Scope2/1, Product/1

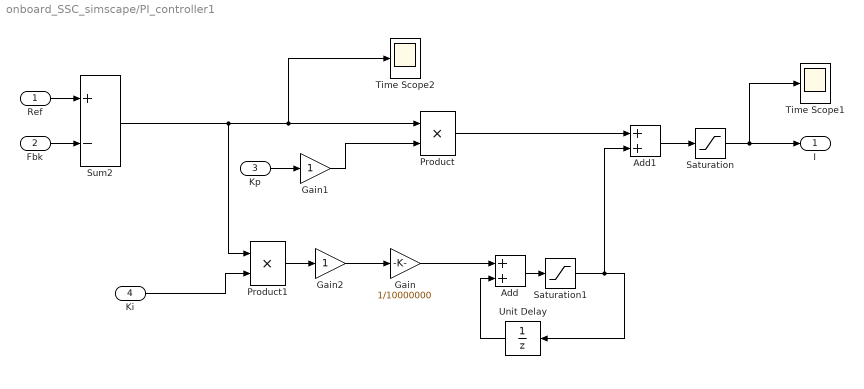
== system onboard_SSC_simscape/PI_controller1 ==
  Ref : Inport
  Fbk : Inport  Port=2
  Kp : Inport  Port=3
  Ki : Inport  Port=4
  Add : Sum
  Add1 : Sum
  Gain : Gain  Gain=1/10000000
  Gain1 : Gain
  Gain2 : Gain
  Product : Product  OutDataTypeStr=Inherit: Same as first input
  Product1 : Product  OutDataTypeStr=Inherit: Same as first input
  Saturation : Saturate  UpperLimit=20  LowerLimit=0  LinearizeAsGain=off  ZeroCross=off
  Saturation1 : Saturate  UpperLimit=30  LowerLimit=-30  LinearizeAsGain=off  ZeroCross=off
  Sum2 : Sum  Inputs=+-
  Time Scope1 : Scope
      settings: TimeUnits=Metric (based on Time Span)  ActiveDisplayYMinimum=10.50458  ActiveDisplayYMaximum=21.05505  YLabel=Amplitude  DataLoggingVariableName=ScopeData5
  Time Scope2 : Scope
      settings: TimeUnits=Metric (based on Time Span)  ActiveDisplayYMinimum=-48.22028  ActiveDisplayYMaximum=227.58003  YLabel=Amplitude  DataLoggingVariableName=ScopeData6
  Unit Delay : UnitDelay  InitialCondition=0.9  SampleTime=-1  HasFrameUpgradeWarning=on
  I : Outport
  wires:
  Fbk/1 -> Sum2/2
  Ref/1 -> Sum2/1
  Product1/1 -> Gain2/1
  Product/1 -> Add1/1
  Gain/1 -> Add/1
  Unit Delay/1 -> Add/2
  Ki/1 -> Product1/2
  Gain2/1 -> Gain/1
  Add1/1 -> Saturation/1
  Saturation/1 -> Time Scope1/1, I/1
  Kp/1 -> Gain1/1
  Gain1/1 -> Product/2
  Sum2/1 -> Product1/1, Time Scope2/1, Product/1
  Add/1 -> Saturation1/1
  Saturation1/1 -> Add1/2, Unit Delay/1

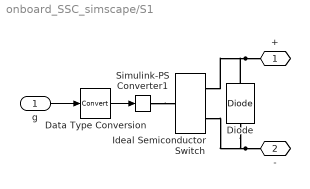
== system onboard_SSC_simscape/S1 ==
  g : Inport
  Data Type Conversion : DataTypeConversion  SaturateOnIntegerOverflow=off  RndMeth=Floor
  Diode : fl_lib/Electrical/Electrical Elements/Diode  Vf=1e-3 V  Ron=0.01 Ohm  Goff=1e-5 1/Ohm  i_specify=off  i_priority=None  i=0 A  i_nominal_specify=off  i_nominal_value=1  i_nominal_unit=A  v_specify=off  v_priority=None  v=0 V  v_nominal_specify=off  v_nominal_value=1  v_nominal_unit=V
  Ideal Semiconductor Switch : ee_lib/Semiconductors & Converters/Ideal Semiconductor Switch  port_option=ee.enum.controlport.ps  Ron=0.1 Ohm  Goff=1e-5 1/Ohm  Vth=0.5 V  diode_param=ee.enum.semiconductors.protectionDiode.external  diode_Vf=1e-3 V  diode_Ron=0.01 Ohm  diode_Goff=1e-5 1/Ohm  diode_C=50e-9 F  diode_iRM=-235 A  diode_iF=300 A  diode_idot=-50 A/us  diode_trr_param=ee.enum.converters.diodetrr.trr_factor  diode_trr_factor=3  diode_trr=15 us  diode_Qrr=1500 s*uA
  Simulink-PS Converter1 : nesl_utility/Simulink-PS Converter  PhysicalDomain=network_engine_domain  SubClassName=ps_input  LeftPortType=input  RightPortType=output  PseudoPeriodic=off  Frequencies=[]  NoiseDistribution=none  NoiseParameters=[]  Unit=1  AffineConversion=off  FilteringAndDerivatives=provide  SimscapeFilterOrder=1  InputFilterTimeConstant=0.001  UdotUserProvided=0
  + : PMIOPort  Side=Left
  - : PMIOPort  Port=2  Side=Right
  wires:
  Data Type Conversion/1 -> Simulink-PS Converter1/1
  g/1 -> Data Type Conversion/1
  connections:
  -/RConn1 -- Diode/LConn1 -- Ideal Semiconductor Switch/RConn2
  +/RConn1 -- Diode/RConn1 -- Ideal Semiconductor Switch/RConn1
  Simulink-PS Converter1/RConn1 -- Ideal Semiconductor Switch/LConn1

== system onboard_SSC_simscape/S2 ==
  g : Inport
  Data Type Conversion : DataTypeConversion  SaturateOnIntegerOverflow=off  RndMeth=Floor
  Diode : fl_lib/Electrical/Electrical Elements/Diode  Vf=1e-3 V  Ron=0.01 Ohm  Goff=1e-5 1/Ohm  i_specify=off  i_priority=None  i=0 A  i_nominal_specify=off  i_nominal_value=1  i_nominal_unit=A  v_specify=off  v_priority=None  v=0 V  v_nominal_specify=off  v_nominal_value=1  v_nominal_unit=V
  Ideal Semiconductor Switch : ee_lib/Semiconductors & Converters/Ideal Semiconductor Switch  port_option=ee.enum.controlport.ps  Ron=0.1 Ohm  Goff=1e-5 1/Ohm  Vth=0.5 V  diode_param=ee.enum.semiconductors.protectionDiode.external  diode_Vf=1e-3 V  diode_Ron=0.01 Ohm  diode_Goff=1e-5 1/Ohm  diode_C=50e-9 F  diode_iRM=-235 A  diode_iF=300 A  diode_idot=-50 A/us  diode_trr_param=ee.enum.converters.diodetrr.trr_factor  diode_trr_factor=3  diode_trr=15 us  diode_Qrr=1500 s*uA
  Simulink-PS Converter1 : nesl_utility/Simulink-PS Converter  PhysicalDomain=network_engine_domain  SubClassName=ps_input  LeftPortType=input  RightPortType=output  PseudoPeriodic=off  Frequencies=[]  NoiseDistribution=none  NoiseParameters=[]  Unit=1  AffineConversion=off  FilteringAndDerivatives=provide  SimscapeFilterOrder=1  InputFilterTimeConstant=0.001  UdotUserProvided=0
  + : PMIOPort  Side=Left
  - : PMIOPort  Port=2  Side=Right
  wires:
  g/1 -> Data Type Conversion/1
  Data Type Conversion/1 -> Simulink-PS Converter1/1
  connections:
  Simulink-PS Converter1/RConn1 -- Ideal Semiconductor Switch/LConn1
  +/RConn1 -- Ideal Semiconductor Switch/RConn1 -- Diode/RConn1
  -/RConn1 -- Ideal Semiconductor Switch/RConn2 -- Diode/LConn1

== system onboard_SSC_simscape/S3 ==
  g : Inport
  Data Type Conversion : DataTypeConversion  SaturateOnIntegerOverflow=off  RndMeth=Floor
  Diode : fl_lib/Electrical/Electrical Elements/Diode  Vf=1e-3 V  Ron=0.01 Ohm  Goff=1e-5 1/Ohm  i_specify=off  i_priority=None  i=0 A  i_nominal_specify=off  i_nominal_value=1  i_nominal_unit=A  v_specify=off  v_priority=None  v=0 V  v_nominal_specify=off  v_nominal_value=1  v_nominal_unit=V
  Ideal Semiconductor Switch : ee_lib/Semiconductors & Converters/Ideal Semiconductor Switch  port_option=ee.enum.controlport.ps  Ron=0.1 Ohm  Goff=1e-5 1/Ohm  Vth=0.5 V  diode_param=ee.enum.semiconductors.protectionDiode.external  diode_Vf=1e-3 V  diode_Ron=0.01 Ohm  diode_Goff=1e-5 1/Ohm  diode_C=50e-9 F  diode_iRM=-235 A  diode_iF=300 A  diode_idot=-50 A/us  diode_trr_param=ee.enum.converters.diodetrr.trr_factor  diode_trr_factor=3  diode_trr=15 us  diode_Qrr=1500 s*uA
  Simulink-PS Converter1 : nesl_utility/Simulink-PS Converter  PhysicalDomain=network_engine_domain  SubClassName=ps_input  LeftPortType=input  RightPortType=output  PseudoPeriodic=off  Frequencies=[]  NoiseDistribution=none  NoiseParameters=[]  Unit=1  AffineConversion=off  FilteringAndDerivatives=provide  SimscapeFilterOrder=1  InputFilterTimeConstant=0.001  UdotUserProvided=0
  + : PMIOPort  Side=Left
  - : PMIOPort  Port=2  Side=Right
  wires:
  g/1 -> Data Type Conversion/1
  Data Type Conversion/1 -> Simulink-PS Converter1/1
  connections:
  Simulink-PS Converter1/RConn1 -- Ideal Semiconductor Switch/LConn1
  +/RConn1 -- Ideal Semiconductor Switch/RConn1 -- Diode/RConn1
  -/RConn1 -- Ideal Semiconductor Switch/RConn2 -- Diode/LConn1

== system onboard_SSC_simscape/S4 ==
  g : Inport
  Data Type Conversion : DataTypeConversion  SaturateOnIntegerOverflow=off  RndMeth=Floor
  Diode : fl_lib/Electrical/Electrical Elements/Diode  Vf=1e-3 V  Ron=0.01 Ohm  Goff=1e-5 1/Ohm  i_specify=off  i_priority=None  i=0 A  i_nominal_specify=off  i_nominal_value=1  i_nominal_unit=A  v_specify=off  v_priority=None  v=0 V  v_nominal_specify=off  v_nominal_value=1  v_nominal_unit=V
  Ideal Semiconductor Switch : ee_lib/Semiconductors & Converters/Ideal Semiconductor Switch  port_option=ee.enum.controlport.ps  Ron=0.1 Ohm  Goff=1e-5 1/Ohm  Vth=0.5 V  diode_param=ee.enum.semiconductors.protectionDiode.external  diode_Vf=1e-3 V  diode_Ron=0.01 Ohm  diode_Goff=1e-5 1/Ohm  diode_C=50e-9 F  diode_iRM=-235 A  diode_iF=300 A  diode_idot=-50 A/us  diode_trr_param=ee.enum.converters.diodetrr.trr_factor  diode_trr_factor=3  diode_trr=15 us  diode_Qrr=1500 s*uA
  Simulink-PS Converter1 : nesl_utility/Simulink-PS Converter  PhysicalDomain=network_engine_domain  SubClassName=ps_input  LeftPortType=input  RightPortType=output  PseudoPeriodic=off  Frequencies=[]  NoiseDistribution=none  NoiseParameters=[]  Unit=1  AffineConversion=off  FilteringAndDerivatives=provide  SimscapeFilterOrder=1  InputFilterTimeConstant=0.001  UdotUserProvided=0
  + : PMIOPort  Side=Left
  - : PMIOPort  Port=2  Side=Right
  wires:
  Data Type Conversion/1 -> Simulink-PS Converter1/1
  g/1 -> Data Type Conversion/1
  connections:
  Diode/LConn1 -- Ideal Semiconductor Switch/RConn2 -- -/RConn1
  Diode/RConn1 -- Ideal Semiconductor Switch/RConn1 -- +/RConn1
  Simulink-PS Converter1/RConn1 -- Ideal Semiconductor Switch/LConn1

== system onboard_SSC_simscape/S5 ==
  g : Inport
  Data Type Conversion : DataTypeConversion  SaturateOnIntegerOverflow=off  RndMeth=Floor
  Diode : fl_lib/Electrical/Electrical Elements/Diode  Vf=1e-3 V  Ron=0.01 Ohm  Goff=1e-5 1/Ohm  i_specify=off  i_priority=None  i=0 A  i_nominal_specify=off  i_nominal_value=1  i_nominal_unit=A  v_specify=off  v_priority=None  v=0 V  v_nominal_specify=off  v_nominal_value=1  v_nominal_unit=V
  Ideal Semiconductor Switch : ee_lib/Semiconductors & Converters/Ideal Semiconductor Switch  port_option=ee.enum.controlport.ps  Ron=0.1 Ohm  Goff=1e-5 1/Ohm  Vth=0.5 V  diode_param=ee.enum.semiconductors.protectionDiode.external  diode_Vf=1e-3 V  diode_Ron=0.01 Ohm  diode_Goff=1e-5 1/Ohm  diode_C=50e-9 F  diode_iRM=-235 A  diode_iF=300 A  diode_idot=-50 A/us  diode_trr_param=ee.enum.converters.diodetrr.trr_factor  diode_trr_factor=3  diode_trr=15 us  diode_Qrr=1500 s*uA
  Simulink-PS Converter1 : nesl_utility/Simulink-PS Converter  PhysicalDomain=network_engine_domain  SubClassName=ps_input  LeftPortType=input  RightPortType=output  PseudoPeriodic=off  Frequencies=[]  NoiseDistribution=none  NoiseParameters=[]  Unit=1  AffineConversion=off  FilteringAndDerivatives=provide  SimscapeFilterOrder=1  InputFilterTimeConstant=0.001  UdotUserProvided=0
  + : PMIOPort  Side=Left
  - : PMIOPort  Port=2  Side=Right
  wires:
  g/1 -> Data Type Conversion/1
  Data Type Conversion/1 -> Simulink-PS Converter1/1
  connections:
  Simulink-PS Converter1/RConn1 -- Ideal Semiconductor Switch/LConn1
  Ideal Semiconductor Switch/RConn1 -- Diode/RConn1 -- +/RConn1
  Ideal Semiconductor Switch/RConn2 -- Diode/LConn1 -- -/RConn1

== system onboard_SSC_simscape/S6 ==
  g : Inport
  Data Type Conversion : DataTypeConversion  SaturateOnIntegerOverflow=off  RndMeth=Floor
  Diode : fl_lib/Electrical/Electrical Elements/Diode  Vf=1e-3 V  Ron=0.01 Ohm  Goff=1e-5 1/Ohm  i_specify=off  i_priority=None  i=0 A  i_nominal_specify=off  i_nominal_value=1  i_nominal_unit=A  v_specify=off  v_priority=None  v=0 V  v_nominal_specify=off  v_nominal_value=1  v_nominal_unit=V
  Ideal Semiconductor Switch : ee_lib/Semiconductors & Converters/Ideal Semiconductor Switch  port_option=ee.enum.controlport.ps  Ron=0.1 Ohm  Goff=1e-5 1/Ohm  Vth=0.5 V  diode_param=ee.enum.semiconductors.protectionDiode.external  diode_Vf=1e-3 V  diode_Ron=0.01 Ohm  diode_Goff=1e-5 1/Ohm  diode_C=50e-9 F  diode_iRM=-235 A  diode_iF=300 A  diode_idot=-50 A/us  diode_trr_param=ee.enum.converters.diodetrr.trr_factor  diode_trr_factor=3  diode_trr=15 us  diode_Qrr=1500 s*uA
  Simulink-PS Converter1 : nesl_utility/Simulink-PS Converter  PhysicalDomain=network_engine_domain  SubClassName=ps_input  LeftPortType=input  RightPortType=output  PseudoPeriodic=off  Frequencies=[]  NoiseDistribution=none  NoiseParameters=[]  Unit=1  AffineConversion=off  FilteringAndDerivatives=provide  SimscapeFilterOrder=1  InputFilterTimeConstant=0.001  UdotUserProvided=0
  + : PMIOPort  Side=Left
  - : PMIOPort  Port=2  Side=Right
  wires:
  Data Type Conversion/1 -> Simulink-PS Converter1/1
  g/1 -> Data Type Conversion/1
  connections:
  Diode/LConn1 -- Ideal Semiconductor Switch/RConn2 -- -/RConn1
  Diode/RConn1 -- Ideal Semiconductor Switch/RConn1 -- +/RConn1
  Simulink-PS Converter1/RConn1 -- Ideal Semiconductor Switch/LConn1

== system onboard_SSC_simscape/S7 ==
  g : Inport
  Data Type Conversion : DataTypeConversion  SaturateOnIntegerOverflow=off  RndMeth=Floor
  Diode : fl_lib/Electrical/Electrical Elements/Diode  Vf=1e-3 V  Ron=0.01 Ohm  Goff=1e-5 1/Ohm  i_specify=off  i_priority=None  i=0 A  i_nominal_specify=off  i_nominal_value=1  i_nominal_unit=A  v_specify=off  v_priority=None  v=0 V  v_nominal_specify=off  v_nominal_value=1  v_nominal_unit=V
  Ideal Semiconductor Switch : ee_lib/Semiconductors & Converters/Ideal Semiconductor Switch  port_option=ee.enum.controlport.ps  Ron=0.1 Ohm  Goff=1e-5 1/Ohm  Vth=0.5 V  diode_param=ee.enum.semiconductors.protectionDiode.external  diode_Vf=1e-3 V  diode_Ron=0.01 Ohm  diode_Goff=1e-5 1/Ohm  diode_C=50e-9 F  diode_iRM=-235 A  diode_iF=300 A  diode_idot=-50 A/us  diode_trr_param=ee.enum.converters.diodetrr.trr_factor  diode_trr_factor=3  diode_trr=15 us  diode_Qrr=1500 s*uA
  Simulink-PS Converter1 : nesl_utility/Simulink-PS Converter  PhysicalDomain=network_engine_domain  SubClassName=ps_input  LeftPortType=input  RightPortType=output  PseudoPeriodic=off  Frequencies=[]  NoiseDistribution=none  NoiseParameters=[]  Unit=1  AffineConversion=off  FilteringAndDerivatives=provide  SimscapeFilterOrder=1  InputFilterTimeConstant=0.001  UdotUserProvided=0
  + : PMIOPort  Side=Left
  - : PMIOPort  Port=2  Side=Right
  wires:
  Data Type Conversion/1 -> Simulink-PS Converter1/1
  g/1 -> Data Type Conversion/1
  connections:
  Diode/LConn1 -- Ideal Semiconductor Switch/RConn2 -- -/RConn1
  Diode/RConn1 -- Ideal Semiconductor Switch/RConn1 -- +/RConn1
  Simulink-PS Converter1/RConn1 -- Ideal Semiconductor Switch/LConn1

== system onboard_SSC_simscape/S8 ==
  g : Inport
  Data Type Conversion : DataTypeConversion  SaturateOnIntegerOverflow=off  RndMeth=Floor
  Diode : fl_lib/Electrical/Electrical Elements/Diode  Vf=1e-3 V  Ron=0.01 Ohm  Goff=1e-5 1/Ohm  i_specify=off  i_priority=None  i=0 A  i_nominal_specify=off  i_nominal_value=1  i_nominal_unit=A  v_specify=off  v_priority=None  v=0 V  v_nominal_specify=off  v_nominal_value=1  v_nominal_unit=V
  Ideal Semiconductor Switch : ee_lib/Semiconductors & Converters/Ideal Semiconductor Switch  port_option=ee.enum.controlport.ps  Ron=0.1 Ohm  Goff=1e-5 1/Ohm  Vth=0.5 V  diode_param=ee.enum.semiconductors.protectionDiode.external  diode_Vf=1e-3 V  diode_Ron=0.01 Ohm  diode_Goff=1e-5 1/Ohm  diode_C=50e-9 F  diode_iRM=-235 A  diode_iF=300 A  diode_idot=-50 A/us  diode_trr_param=ee.enum.converters.diodetrr.trr_factor  diode_trr_factor=3  diode_trr=15 us  diode_Qrr=1500 s*uA
  Simulink-PS Converter1 : nesl_utility/Simulink-PS Converter  PhysicalDomain=network_engine_domain  SubClassName=ps_input  LeftPortType=input  RightPortType=output  PseudoPeriodic=off  Frequencies=[]  NoiseDistribution=none  NoiseParameters=[]  Unit=1  AffineConversion=off  FilteringAndDerivatives=provide  SimscapeFilterOrder=1  InputFilterTimeConstant=0.001  UdotUserProvided=0
  + : PMIOPort  Side=Left
  - : PMIOPort  Port=2  Side=Right
  wires:
  g/1 -> Data Type Conversion/1
  Data Type Conversion/1 -> Simulink-PS Converter1/1
  connections:
  Simulink-PS Converter1/RConn1 -- Ideal Semiconductor Switch/LConn1
  +/RConn1 -- Ideal Semiconductor Switch/RConn1 -- Diode/RConn1
  -/RConn1 -- Ideal Semiconductor Switch/RConn2 -- Diode/LConn1

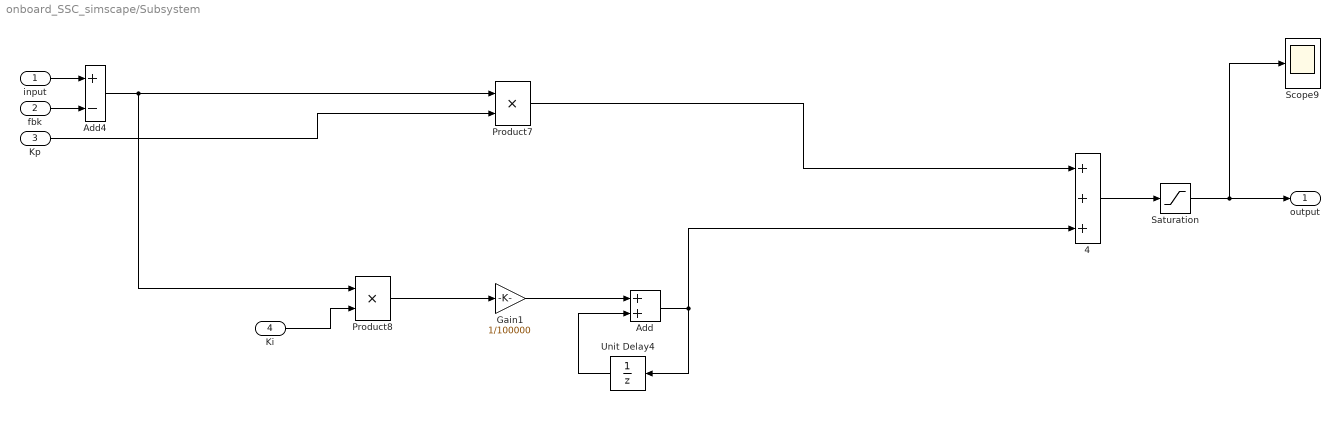
== system onboard_SSC_simscape/Subsystem ==
  input : Inport
  fbk : Inport  Port=2
  Kp : Inport  Port=3
  Ki : Inport  Port=4
  4 : Sum  Inputs=+++
  Add : Sum
  Add4 : Sum  Inputs=+-
  Gain1 : Gain  Gain=1/100000
  Product7 : Product  OutDataTypeStr=Inherit: Same as first input
  Product8 : Product  OutDataTypeStr=Inherit: Same as first input
  Saturation : Saturate  UpperLimit=450  LowerLimit=-450  LinearizeAsGain=off  ZeroCross=off
  Scope9 : Scope
      settings: ActiveDisplayYMinimum=-562.5  ActiveDisplayYMaximum=562.5  DataLoggingVariableName=ScopeData2
  Unit Delay4 : UnitDelay  SampleTime=-1  HasFrameUpgradeWarning=on
  output : Outport
  wires:
  Kp/1 -> Product7/2
  Product7/1 -> 4/1
  input/1 -> Add4/1
  fbk/1 -> Add4/2
  Gain1/1 -> Add/1
  Add4/1 -> Product7/1, Product8/1
  Unit Delay4/1 -> Add/2
  Product8/1 -> Gain1/1
  Add/1 -> Unit Delay4/1, 4/3
  Ki/1 -> Product8/2
  4/1 -> Saturation/1
  Saturation/1 -> Scope9/1, output/1

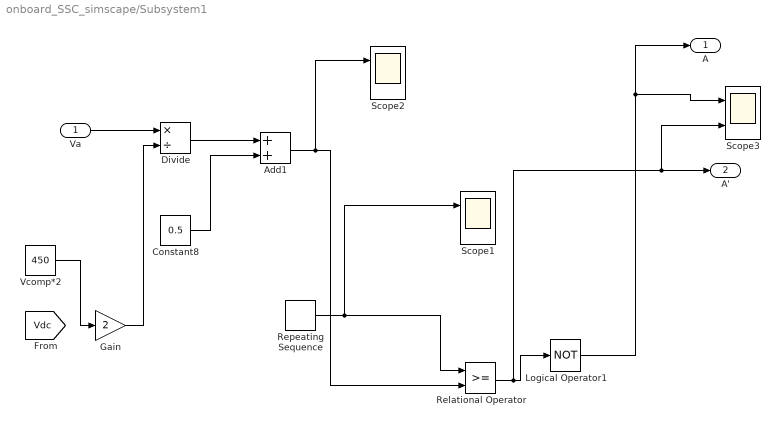
== system onboard_SSC_simscape/Subsystem1 ==
  Va : Inport
  Add1 : Sum
  Constant8 : Constant  Value=0.5
  Divide : Product  Inputs=*/
  Gain : Gain  Gain=2
  Logical Operator1 : Logic  Operator=NOT  AllPortsSameDT=off  OutDataTypeStr=boolean
  Relational Operator : RelationalOperator  OutDataTypeStr=boolean  ZeroCross=off  InputSameDT=off
  Repeating Sequence : simulink/Sources/Repeating Sequence  rep_seq_t=[0 1/30000/2 1/30000]  rep_seq_y=[0 1 0]
  Scope1 : Scope  NumInputPorts=2
      settings: ActiveDisplayYMinimum=0.28433  ActiveDisplayYMaximum=0.71367  DataLoggingVariableName=ScopeData3
  Scope2 : Scope  NumInputPorts=2
      settings: ActiveDisplayYMinimum=-1.10476173144655E+9  ActiveDisplayYMaximum=9.94285024582082E+9
  Scope3 : Scope  NumInputPorts=2
      settings: ActiveDisplayYMinimum=0.40709  ActiveDisplayYMaximum=0.54786  DataLoggingVariableName=ScopeData2
  Vcomp*2 : Constant  Value=450
  A : Outport
  A' : Outport  Port=2
  wires:
  Va/1 -> Divide/1
  Divide/1 -> Add1/1
  Add1/1 -> Scope2/1, Relational Operator/2
  Constant8/1 -> Add1/2
  Repeating Sequence/1 -> Scope1/1, Relational Operator/1
  Logical Operator1/1 -> Scope3/1, A/1
  Relational Operator/1 -> Scope3/2, A'/1, Logical Operator1/1
  Gain/1 -> Divide/2
  Vcomp*2/1 -> Gain/1

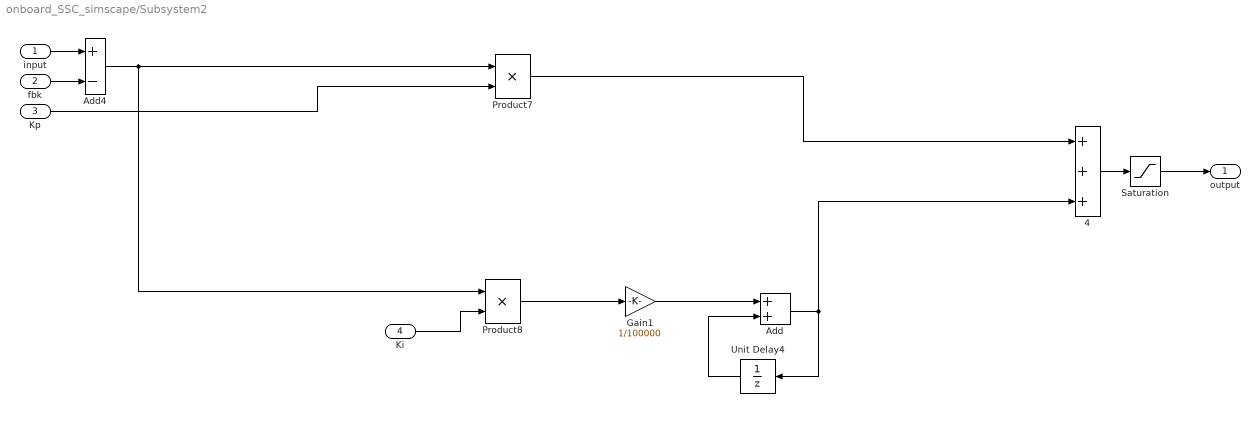
== system onboard_SSC_simscape/Subsystem2 ==
  input : Inport
  fbk : Inport  Port=2
  Kp : Inport  Port=3
  Ki : Inport  Port=4
  4 : Sum  Inputs=+++
  Add : Sum
  Add4 : Sum  Inputs=+-
  Gain1 : Gain  Gain=1/100000
  Product7 : Product  OutDataTypeStr=Inherit: Same as first input
  Product8 : Product  OutDataTypeStr=Inherit: Same as first input
  Saturation : Saturate  UpperLimit=450  LowerLimit=-450  LinearizeAsGain=off  ZeroCross=off
  Unit Delay4 : UnitDelay  SampleTime=-1  HasFrameUpgradeWarning=on
  output : Outport
  wires:
  Kp/1 -> Product7/2
  Product7/1 -> 4/1
  input/1 -> Add4/1
  fbk/1 -> Add4/2
  4/1 -> Saturation/1
  Add4/1 -> Product7/1, Product8/1
  Ki/1 -> Product8/2
  Unit Delay4/1 -> Add/2
  Product8/1 -> Gain1/1
  Add/1 -> Unit Delay4/1, 4/3
  Gain1/1 -> Add/1
  Saturation/1 -> output/1
